simulink model "giaeb_ut"  (Simulink 8.1)
settings: Solver=FixedStepDiscrete  StartTime=0.0  StopTime=10.0  FixedStep=0.005  RelTol=1e-3
libraries: siltestlib x10, idiada_lib x4, giaeb x1
settings Model: Creator=xsellart  LastModifiedBy=AT015555
settings DataIOCC: SignalLoggingSaveFormat=Dataset
settings OptimizationCC: ExpressionDepthLimit=128
settings DebuggingCC: FcnCallInpInsideContextMsg=EnableAllAsError
settings GRTTargetCC: CombineOutputUpdateFcns=on  GRTInterface=off

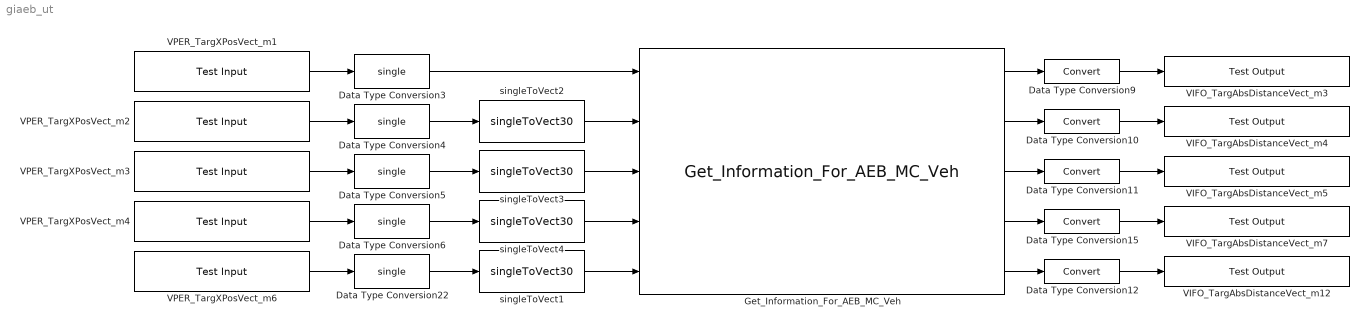
== system giaeb_ut ==
  Data Type Conversion{9..12,15} (5 alike) : DataTypeConversion
  Data Type Conversion{3..6,22} (5 alike) : DataTypeConversion  OutDataTypeStr=single
  Get_Information_For_AEB_MC_Veh : giaeb/Get_Information_For_AEB_MC_Veh
  VIFO_TargAbsDistanceVect_m12 : siltestlib/Test Output  varname=NIFO_AEBMCLongAccel_mps2  sampletime=-1
  VIFO_TargAbsDistanceVect_m3 : siltestlib/Test Output  varname=NIFO_AEBTargetVehRelSpeedX_mps  sampletime=-1
  VIFO_TargAbsDistanceVect_m4 : siltestlib/Test Output  varname=NIFO_AEBMCVehXPosition_m  sampletime=-1
  VIFO_TargAbsDistanceVect_m5 : siltestlib/Test Output  varname=NIFO_AEBTargetVehAssigned_flg  sampletime=-1
  VIFO_TargAbsDistanceVect_m7 : siltestlib/Test Output  varname=NIFO_AEBMCVehId_num  sampletime=-1
  VPER_TargXPosVect_m1 : siltestlib/Test Input  varname=VIFO_AEBMCTTargetId_num  sampletime=0.005
  VPER_TargXPosVect_m2 : siltestlib/Test Input  varname=VPER_TargXPosVect30_m  sampletime=0.005
  VPER_TargXPosVect_m3 : siltestlib/Test Input  varname=VIFO_TargVehRelSpdXVect30_mps  sampletime=0.005
  VPER_TargXPosVect_m4 : siltestlib/Test Input  varname=VPER_TargIdVect30_num  sampletime=0.005
  VPER_TargXPosVect_m6 : siltestlib/Test Input  varname=VIFO_TargAccelXVect30_mps2  sampletime=0.005
  singleToVect{1..4} (4 alike) : idiada_lib/singleToVect30
  wires:
  VPER_TargXPosVect_m1/1 -> Data Type Conversion3/1
  Data Type Conversion3/1 -> Get_Information_For_AEB_MC_Veh/1
  VPER_TargXPosVect_m2/1 -> Data Type Conversion4/1
  Data Type Conversion4/1 -> singleToVect2/1
  VPER_TargXPosVect_m3/1 -> Data Type Conversion5/1
  Data Type Conversion5/1 -> singleToVect3/1
  VPER_TargXPosVect_m4/1 -> Data Type Conversion6/1
  Data Type Conversion6/1 -> singleToVect4/1
  Get_Information_For_AEB_MC_Veh/1 -> Data Type Conversion9/1
  Data Type Conversion9/1 -> VIFO_TargAbsDistanceVect_m3/1
  Get_Information_For_AEB_MC_Veh/2 -> Data Type Conversion10/1
  Data Type Conversion10/1 -> VIFO_TargAbsDistanceVect_m4/1
  Get_Information_For_AEB_MC_Veh/3 -> Data Type Conversion11/1
  Data Type Conversion11/1 -> VIFO_TargAbsDistanceVect_m5/1
  Data Type Conversion12/1 -> VIFO_TargAbsDistanceVect_m12/1
  singleToVect2/1 -> Get_Information_For_AEB_MC_Veh/2
  singleToVect3/1 -> Get_Information_For_AEB_MC_Veh/3
  singleToVect4/1 -> Get_Information_For_AEB_MC_Veh/4
  Get_Information_For_AEB_MC_Veh/5 -> Data Type Conversion12/1
  Data Type Conversion15/1 -> VIFO_TargAbsDistanceVect_m7/1
  Get_Information_For_AEB_MC_Veh/4 -> Data Type Conversion15/1
  VPER_TargXPosVect_m6/1 -> Data Type Conversion22/1
  Data Type Conversion22/1 -> singleToVect1/1
  singleToVect1/1 -> Get_Information_For_AEB_MC_Veh/5
